simulink model "Thermoacoustic_Model"  (R2019a)
settings: Solver=VariableStepAuto  StartTime=0.0  StopTime=100  RelTol=1e-3
model workspace (MAT data in the model file):
  P_a = 0
  Param = Simulink.Parameter
  Param.Value = 0
  Param.DataType = 'double'
  Param.Dimensions = [1 1]
  freq_k = 0
settings Model: OrderedModelArguments=off  Creator=bbraunj  LastModifiedBy=bbraunj

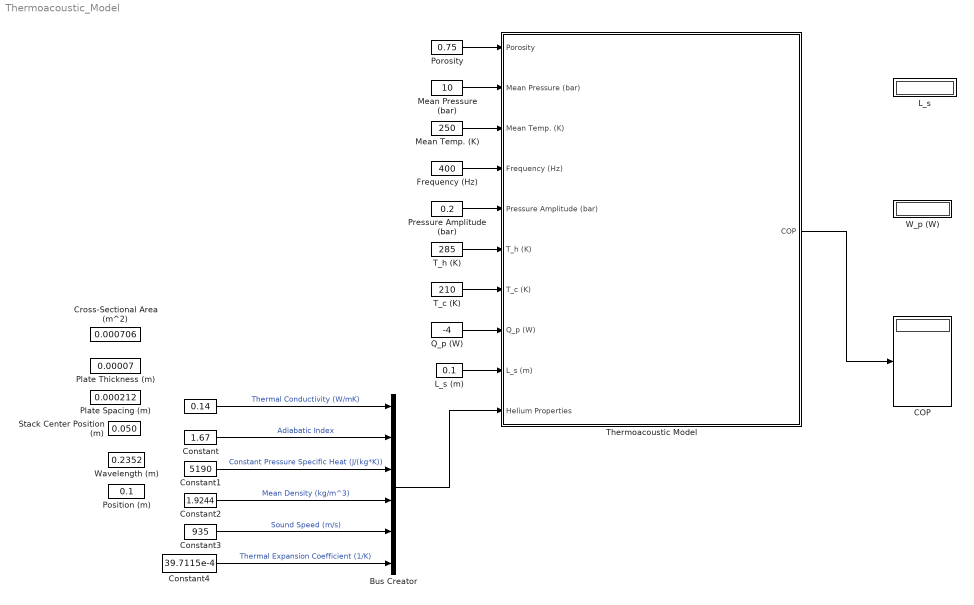
== system Thermoacoustic_Model ==
  " " : Constant  Value=0.14
  Bus Creator : BusCreator  Inputs=6
  COP : Display
  Constant : Constant  Value=1.67
  Constant1 : Constant  Value=5190
  Constant2 : Constant  Value=1.9244
  Constant3 : Constant  Value=935
  Constant4 : Constant  Value=39.7115e-4
  Cross-Sectional Area (m^2) : Constant  Value=0.000706
  Frequency (Hz) : Constant  Value=400
  L_s : Display
  L_s (m) : Constant  Value=0.1
  Mean Pressure (bar) : Constant  Value=10
  Mean Temp. (K) : Constant  Value=250
  Plate Spacing (m) : Constant  Value=0.000212
  Plate Thickness (m) : Constant  Value=0.00007
  Porosity : Constant  Value=0.75
  Position (m) : Constant  Value=0.1
  Pressure Amplitude (bar) : Constant  Value=0.2
  "Q_p (W) " : Constant  Value=-4
  Stack Center Position (m) : Constant  Value=0.050
  T_c (K) : Constant  Value=210
  T_h (K) : Constant  Value=285
  Thermoacoustic Model : Subsystem
  W_p (W) : Display
  Wavelength (m) : Constant  Value=0.2352
  wires:
  Porosity/1 -> Thermoacoustic Model/1(Porosity)
  Mean Pressure (bar)/1 -> Thermoacoustic Model/2(Mean Pressure (bar))
  Mean Temp. (K)/1 -> Thermoacoustic Model/3(Mean Temp. (K))
  Frequency (Hz)/1 -> Thermoacoustic Model/4(Frequency (Hz))
  Pressure Amplitude (bar)/1 -> Thermoacoustic Model/5(Pressure Amplitude (bar))
  T_h (K)/1 -> Thermoacoustic Model/6(T_h (K))
  T_c (K)/1 -> Thermoacoustic Model/7(T_c (K))
  " "/1 -> Bus Creator/1  "Thermal Conductivity (W/mK)"
  Constant/1 -> Bus Creator/2  "Adiabatic Index"
  Constant1/1 -> Bus Creator/3  "Constant Pressure Specific Heat (J/(kg*K))"
  Constant2/1 -> Bus Creator/4  "Mean Density (kg/m^3)"
  Constant3/1 -> Bus Creator/5  "Sound Speed (m/s)"
  Constant4/1 -> Bus Creator/6  "Thermal Expansion Coefficient (1/K)"
  Bus Creator/1 -> Thermoacoustic Model/10(Helium Properties)
  ? -> L_s/1
  ? -> W_p (W)/1
  Thermoacoustic Model/1(COP) -> COP/1
  "Q_p (W) "/1 -> Thermoacoustic Model/8(Q_p (W))
  L_s (m)/1 -> Thermoacoustic Model/9("L_s (m) ")

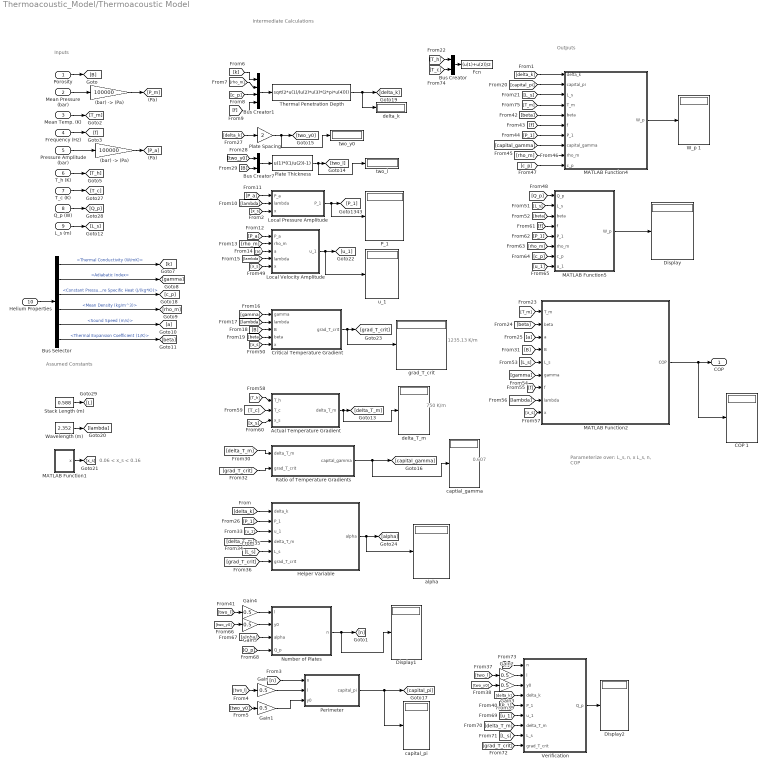
== system Thermoacoustic_Model/Thermoacoustic Model ==
  note: 0.06 < x_s < 0.16
  note: Inputs
  note: Outputs
  note: Intermediate Calculations
  note: 1235.13 K/m
  note: 750 K/m
  note: 0.607
  note: Assumed Constants
  note: Parameterize over:
      | L_s, n, x
      | L_s, n, COP
  Porosity : Inport
  Mean Pressure (bar) : Inport  Port=2
  Mean Temp. (K) : Inport  Port=3
  Frequency (Hz) : Inport  Port=4
  Pressure Amplitude (bar) : Inport  Port=5
  T_h (K) : Inport  Port=6
  T_c (K) : Inport  Port=7
  Q_p (W) : Inport  Port=8
  "L_s (m) " : Inport  Port=9
  Helium Properties : Inport  Port=10
  "(bar) -> (Pa)" : Gain  Gain=100000
  "(bar) -> (Pa) " : Gain  Gain=100000
  Actual Temperature Gradient : MATLAB Function  TreatAsAtomicUnit=on
  Bus Creator : BusCreator  Inputs=2
  Bus Creator1 : BusCreator  Inputs=4
  Bus Creator7 : BusCreator  Inputs=2
  Bus Selector : BusSelector  OutputSignals=Thermal Conductivity (W/mK),Adiabatic Index,Constant Pressure Specific Heat (J/(kg*K)),Mean Density (kg/m^3),Sound Speed (m/s),Thermal Expansion Coefficient (1/K)
  COP 1 : Display
  Critical Temperature Gradient : MATLAB Function  TreatAsAtomicUnit=on
  Display : Display
  Display1 : Display
  Display2 : Display
  Fcn : Fcn  Expr=(u(1)+u(2))/2
  Gain{,1..5} (6 alike) : Gain  Gain=0.5
  Helper Variable : MATLAB Function  TreatAsAtomicUnit=on
  Local Pressure Amplitude : MATLAB Function  TreatAsAtomicUnit=on
  Local Velocity Amplitude : MATLAB Function  TreatAsAtomicUnit=on
  MATLAB Function1 : MATLAB Function  TreatAsAtomicUnit=on
  MATLAB Function2 : MATLAB Function  TreatAsAtomicUnit=on
  MATLAB Function4 : MATLAB Function  TreatAsAtomicUnit=on
  MATLAB Function5 : MATLAB Function  TreatAsAtomicUnit=on
  Number of Plates : MATLAB Function  TreatAsAtomicUnit=on
  P_1 : Display
  Perimeter : MATLAB Function  TreatAsAtomicUnit=on
  Plate Spacing : Gain  Gain=2
  "Plate Thickness " : Fcn  Expr=u(1)*((1/u(2))-1)
  Ratio of Temperature Gradients : MATLAB Function  TreatAsAtomicUnit=on
  Stack Length (m) : Constant  Value=0.588
  Thermal Penetration Depth : Fcn  Expr=sqrt(2*u(1)/(u(2)*u(3)*(2*pi*u(4))))
  Verification : MATLAB Function  TreatAsAtomicUnit=on
  W_p 1 : Display
  Wavelength (m) : Constant  Value=2.352
  alpha : Display
  capital_pi : Display
  captial_gamma : Display
  delta_T_m : Display
  delta_k : Display
  grad_T_crit : Display
  two_l : Display
  two_y0 : Display
  u_1 : Display
  COP : Outport
  wires:
  Mean Temp. (K)/1 -> [T_m]
  "L_s (m) "/1 -> [L_s]
  T_h (K)/1 -> [T_h]
  Frequency (Hz)/1 -> [f]
  Porosity/1 -> [B]
  Thermal Penetration Depth/1 -> delta_k/1, [delta_k]
  Bus Creator1/1 -> Thermal Penetration Depth/1
  [k] -> Bus Creator1/1
  [rho_m] -> Bus Creator1/2
  [c_p] -> Bus Creator1/3
  [f] -> Bus Creator1/4
  Critical Temperature Gradient/1(grad_T_crit) -> grad_T_crit/1, [grad_T_crit]
  T_c (K)/1 -> [T_c]
  Q_p (W)/1 -> [Q_p]
  Helium Properties/1 -> Bus Selector/1
  Bus Selector/2 -> [gamma]  "<Adiabatic Index>"
  Bus Selector/3 -> [c_p]  "<Constant Pressure Specific Heat (J/(kg*K))>"
  Stack Length (m)/1 -> [L]
  Wavelength (m)/1 -> [lambda]
  [delta_k] -> Plate Spacing/1
  Plate Spacing/1 -> two_y0/1, [two_y0]
  [two_y0] -> Bus Creator7/1
  [B] -> Bus Creator7/2
  Bus Creator7/1 -> "Plate Thickness "/1
  "Plate Thickness "/1 -> two_l/1, [two_l]
  Bus Selector/1 -> [k]  "<Thermal Conductivity (W/mK)>"
  Bus Selector/4 -> [rho_m]  "<Mean Density (kg/m^3)>"
  Bus Selector/5 -> [a]  "<Sound Speed (m/s)>"
  Bus Selector/6 -> [beta]  "<Thermal Expansion Coefficient (1/K)>"
  MATLAB Function1/1(x) -> [x_s]
  [x_s] -> Local Pressure Amplitude/3(x)
  [lambda] -> Local Pressure Amplitude/2(lambda)
  [P_a] -> Local Pressure Amplitude/1(P_a)
  Local Pressure Amplitude/1(P_1) -> P_1/1, [P_1]
  [P_a] -> Local Velocity Amplitude/1(P_a)
  [rho_m] -> Local Velocity Amplitude/2(rho_m)
  [a] -> Local Velocity Amplitude/3(a)
  [lambda] -> Local Velocity Amplitude/4(lambda)
  [x_s] -> Local Velocity Amplitude/5(x)
  Local Velocity Amplitude/1(u_1) -> u_1/1, [u_1]
  [gamma] -> Critical Temperature Gradient/1(gamma)
  [lambda] -> Critical Temperature Gradient/2(lambda)
  [B] -> Critical Temperature Gradient/3(B)
  [beta] -> Critical Temperature Gradient/4(beta)
  [x_s] -> Critical Temperature Gradient/5(x)
  [grad_T_crit] -> Ratio of Temperature Gradients/2(grad_T_crit)
  [delta_T_m] -> Ratio of Temperature Gradients/1(delta_T_m)
  Ratio of Temperature Gradients/1(capital_gamma) -> [capital_gamma], captial_gamma/1
  [B] -> MATLAB Function2/4(B)
  [f] -> MATLAB Function2/7(f)
  [a] -> MATLAB Function2/3(a)
  [lambda] -> MATLAB Function2/8(lambda)
  [L_s] -> MATLAB Function2/5(L_s)
  [x_s] -> MATLAB Function2/9(x)
  [T_m] -> MATLAB Function2/1(T_m)
  [gamma] -> MATLAB Function2/6(gamma)
  [beta] -> MATLAB Function2/2(beta)
  MATLAB Function2/1(COP) -> COP/1, COP 1/1
  [T_c] -> Actual Temperature Gradient/2(T_c)
  [x_s] -> Actual Temperature Gradient/3(x_s)
  Actual Temperature Gradient/1(delta_T_m) -> delta_T_m/1, [delta_T_m]
  [T_h] -> Actual Temperature Gradient/1(T_h)
  [c_p] -> MATLAB Function4/10(c_p)
  [P_1] -> MATLAB Function4/7(P_1)
  [beta] -> MATLAB Function4/5(beta)
  [capital_pi] -> MATLAB Function4/2(capital_pi)
  [capital_gamma] -> MATLAB Function4/8(capital_gamma)
  [delta_k] -> MATLAB Function4/1(delta_k)
  [L_s] -> MATLAB Function4/3(L_s)
  [rho_m] -> MATLAB Function4/9(rho_m)
  [f] -> MATLAB Function4/6(f)
  MATLAB Function4/1(W_p) -> W_p 1/1
  [Q_p] -> MATLAB Function5/1(Q_p)
  [L_s] -> MATLAB Function5/2(L_s)
  [beta] -> MATLAB Function5/3(beta)
  [f] -> MATLAB Function5/4(f)
  [P_1] -> MATLAB Function5/5(P_1)
  [rho_m] -> MATLAB Function5/6(rho_m)
  [c_p] -> MATLAB Function5/7(c_p)
  [u_1] -> MATLAB Function5/8(u_1)
  MATLAB Function5/1(W_p) -> Display/1
  [delta_k] -> Helper Variable/1(delta_k)
  [P_1] -> Helper Variable/2(P_1)
  [u_1] -> Helper Variable/3(u_1)
  [delta_T_m] -> Helper Variable/4(delta_T_m)
  [grad_T_crit] -> Helper Variable/6(grad_T_crit)
  Helper Variable/1(alpha) -> alpha/1, [alpha]
  [two_l] -> Gain4/1
  Gain4/1 -> Number of Plates/1(l)
  [two_y0] -> Gain5/1
  Gain5/1 -> Number of Plates/2(y0)
  [alpha] -> Number of Plates/3(alpha)
  [Q_p] -> Number of Plates/4(Q_p)
  Number of Plates/1(n) -> Display1/1, [n]
  Pressure Amplitude (bar)/1 -> "(bar) -> (Pa)"/1
  "(bar) -> (Pa)"/1 -> [P_a]
  Mean Pressure (bar)/1 -> "(bar) -> (Pa) "/1
  "(bar) -> (Pa) "/1 -> [P_m]
  [L_s] -> Helper Variable/5(L_s)
  [n] -> Perimeter/1(n)
  Gain/1 -> Perimeter/2(l)
  [two_l] -> Gain/1
  Perimeter/1(capital_pi) -> capital_pi/1, [capital_pi]
  [two_y0] -> Gain1/1
  Gain1/1 -> Perimeter/3(y0)
  [two_l] -> Gain2/1
  [two_y0] -> Gain3/1
  Gain2/1 -> Verification/2(l)
  Gain3/1 -> Verification/3(y0)
  [delta_k] -> Verification/4(delta_k)
  [P_1] -> Verification/5(P_1)
  [u_1] -> Verification/6(u_1)
  [delta_T_m] -> Verification/7(delta_T_m)
  [L_s] -> Verification/8(L_s)
  [grad_T_crit] -> Verification/9(grad_T_crit)
  [n] -> Verification/1(n)
  Verification/1(Q_p) -> Display2/1
  Bus Creator/1 -> Fcn/1
  [T_h] -> Bus Creator/1
  [T_c] -> Bus Creator/2
  [T_m] -> MATLAB Function4/4(T_m)

== matlab function Thermoacoustic_Model/Thermoacoustic Model/MATLAB Function1 ==
  data: x output
function x = fcn()
x = [0.06:0.02:0.16];

== matlab function Thermoacoustic_Model/Thermoacoustic Model/Local Pressure Amplitude ==
  data: P_a input; P_1 output; lambda input; x input
function P_1 = fcn(P_a, lambda, x)
P_1 = P_a*cos((2*pi/lambda)*x);

== matlab function Thermoacoustic_Model/Thermoacoustic Model/Local Velocity Amplitude ==
  data: P_a input; u_1 output; rho_m input; a input; lambda input; x input
function u_1 = fcn(P_a, rho_m, a, lambda, x)
u_1 = (P_a/(rho_m*a))*sin((2*pi/lambda)*x);

== matlab function Thermoacoustic_Model/Thermoacoustic Model/Critical Temperature Gradient ==
  data: gamma input; grad_T_crit output; lambda input; B input; beta input; x input
function grad_T_crit = fcn(gamma, lambda, B, beta, x)
k = 2*pi/lambda;
grad_T_crit = ((gamma-1)*k*B/beta)*cot(k*x);

== matlab function Thermoacoustic_Model/Thermoacoustic Model/Ratio of Temperature Gradients ==
  data: delta_T_m input; capital_gamma output; grad_T_crit input
function capital_gamma = fcn(delta_T_m, grad_T_crit)
capital_gamma = zeros(size(grad_T_crit));
for idx = 1:numel(grad_T_crit)
    capital_gamma(idx) = delta_T_m(idx)/grad_T_crit(idx);
end

== matlab function Thermoacoustic_Model/Thermoacoustic Model/MATLAB Function2 ==
  data: T_m input; COP output; beta input; a input; B input; L_s input; gamma input; f input; lambda input; x input
function COP = fcn(T_m, beta, a, B, L_s, gamma, f, lambda, x)
COP = (T_m*beta*a/(B*L_s*(gamma-1)*(2*pi*f)))*tan((2*pi/lambda)*x);

== matlab function Thermoacoustic_Model/Thermoacoustic Model/Actual Temperature Gradient ==
  data: T_h input; delta_T_m output; T_c input; x_s input
function delta_T_m = fcn(T_h, T_c, x_s)
for idx = 1:numel(x_s)
    x_s(idx) = 1/x_s(idx);
end
delta_T_m = (T_h - T_c)*x_s;

== matlab function Thermoacoustic_Model/Thermoacoustic Model/MATLAB Function4 ==
  data: delta_k input; W_p output; capital_pi input; L_s input; T_m input; beta input; f input; P_1 input; capital_gamma input; rho_m input; c_p input
function W_p = fcn(delta_k, capital_pi, L_s, T_m, beta, f, P_1, capital_gamma, rho_m, c_p)
W_p = zeros(size(P_1));
for idx = 1:numel(P_1)
    W_p(idx) = (delta_k*capital_pi(idx)*L_s*T_m*(beta^2)*(2*pi*f)/(4*rho_m*c_p))*(P_1(idx)^2)*((capital_gamma(idx)/L_s)-1);
end

== matlab function Thermoacoustic_Model/Thermoacoustic Model/MATLAB Function5 ==
  data: Q_p input; W_p output; L_s input; beta input; f input; P_1 input; rho_m input; c_p input; u_1 input
function W_p = fcn(Q_p, L_s, beta, f, P_1, rho_m, c_p, u_1)
W_p = zeros(size(P_1));
for idx = 1:numel(P_1)
    W_p(idx) = -Q_p*L_s*beta*(2*pi*f)*P_1(idx)/( rho_m*c_p*u_1(idx) );
end

== matlab function Thermoacoustic_Model/Thermoacoustic Model/Helper Variable ==
  data: delta_k input; alpha output; P_1 input; u_1 input; delta_T_m input; L_s input; grad_T_crit input
function alpha = fcn(delta_k, P_1, u_1, delta_T_m, L_s, grad_T_crit)
alpha = zeros(size(P_1));
for idx = 1:numel(P_1)
    alpha(idx) = delta_k*P_1(idx)*u_1(idx)*( delta_T_m(idx)/(L_s*grad_T_crit(idx)) - 1);
end

== matlab function Thermoacoustic_Model/Thermoacoustic Model/Number of Plates ==
  data: l input; n output; y0 input; alpha input; Q_p input
function n = fcn(l, y0, alpha, Q_p)
n = zeros(size(alpha));
for idx = 1:numel(alpha)
    n(idx) = (y0 + sqrt(y0^2 - 4*(l+y0)*(Q_p/alpha(idx))))/(2*(l+y0));
end

== matlab function Thermoacoustic_Model/Thermoacoustic Model/Perimeter ==
  data: n input; capital_pi output; l input; y0 input
function capital_pi = fcn(n, l, y0)
capital_pi = zeros(size(n));
for idx = 1:numel(capital_pi)
    capital_pi(idx) = 4*n(idx)*l + 4*(n(idx)-1)*y0;
end

== matlab function Thermoacoustic_Model/Thermoacoustic Model/Verification ==
  data: n input; Q_p output; l input; y0 input; delta_k input; P_1 input; u_1 input; delta_T_m input; L_s input; grad_T_crit input
function Q_p = fcn(n, l, y0, delta_k, P_1, u_1, delta_T_m, L_s, grad_T_crit)
Q_p = zeros(size(n));
for idx = 1:numel(n)
    Q_p(idx) = -n(idx)*(n(idx)*(l+y0)-y0)*delta_k*P_1(idx)*u_1(idx)*( delta_T_m(idx)/(L_s*grad_T_crit(idx)) - 1);
end
